simulink model "ANCbyFxLMS"  (R2024a)
settings: Solver=FixedStepDiscrete  StartTime=0.0  StopTime=1000000  RelTol=1e-3
settings Model: Creator=chenxinzhang  LastModifiedBy=chenxinzhang
settings SolverCC: AlgebraicLoopSolver=TrustRegion  AutoInsertRateTranBlk=on
settings DataIOCC: LimitDataPoints=on  SaveOutput=off  SignalLogging=off  SaveTime=off
settings OptimizationCC: LifeSpan=inf
settings DebuggingCC: AlgebraicLoopMsg=error  SingleTaskRateTransMsg=error  UnconnectedInputMsg=warning  UnconnectedOutputMsg=warning  UnconnectedLineMsg=warning  AllowSymbolicDim=off  SFUnexpectedBacktrackingDiag=warning  SFNoUnconditionalDefaultTransitionDiag=warning  SFExecutionAtInitializationDiag=none  ArithmeticOperatorsInVariantConditions=warning
settings ModelReferenceCC: EnableRefExpFcnMdlSchedulingChecks=on
settings SFSimCC: SimUseLocalCustomCode=off  CustomCodeUndefinedFunction=UseInterfaceOnly
settings RTWCC: RTWUseLocalCustomCode=off  GPUComputeCapability=3.5
settings CodeAppCC: StateflowObjectComments=on
settings GRTTargetCC: TargetLangStandard=C89/C90 (ANSI)
settings ConfigComp: CovMetricSettings=dw  CovSaveCumulativeToWorkspaceVar=on  CovSaveSingleToWorkspaceVar=on  CovExternalEMLEnable=off  CovSFcnEnable=off

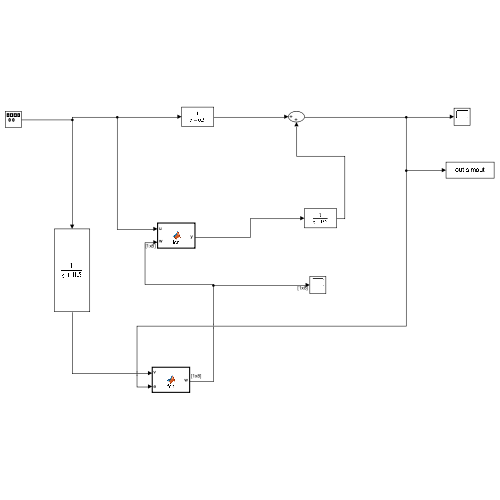
[thumbnail: Simulink's stored preview of the top-level diagram]
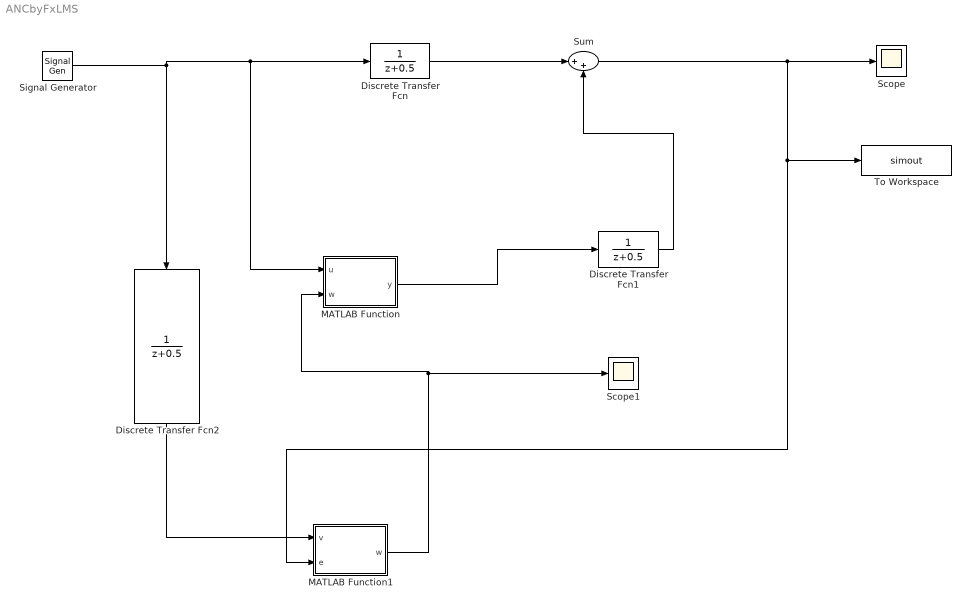
== system ANCbyFxLMS ==
  Discrete Transfer Fcn : DiscreteTransferFcn  Numerator=[0 1]
  Discrete Transfer Fcn1 : DiscreteTransferFcn  Numerator=[0 1]
  Discrete Transfer Fcn2 : DiscreteTransferFcn  Numerator=[0 1]
  MATLAB Function : MATLAB Function  TreatAsAtomicUnit=on
  MATLAB Function1 : MATLAB Function  TreatAsAtomicUnit=on
  Scope : Scope
  Scope1 : Scope
  Signal Generator : SignalGenerator  Frequency=10  Units=rad/sec
  Sum : Sum  Inputs=|++
  To Workspace : ToWorkspace  VariableName=simout  SaveFormat=Timeseries  SampleTime=-1
  wires:
  Signal Generator/1 -> Discrete Transfer Fcn2/1, MATLAB Function/1(u), Discrete Transfer Fcn/1
  Discrete Transfer Fcn/1 -> Sum/1
  Discrete Transfer Fcn1/1 -> Sum/2
  Sum/1 -> To Workspace/1, MATLAB Function1/2(e), Scope/1
  Discrete Transfer Fcn2/1 -> MATLAB Function1/1(v)
  MATLAB Function/1(y) -> Discrete Transfer Fcn1/1
  MATLAB Function1/1(w) -> Scope1/1, MATLAB Function/2(w)

== matlab function ANCbyFxLMS/MATLAB Function ==
  data: u input; y output; w input
function y = fcn(u, w)
%#codegen
persistent xbuf

if isempty(xbuf)
    xbuf = zeros(1,8);
end

xbuf(2:8) = xbuf(1:7);
xbuf(1) = u;

y = w * xbuf.';

if ~isfinite(y)
    y = 0;
elseif y > 1e3
    y = 1e3;
elseif y < -1e3
    y = -1e3;
end

== matlab function ANCbyFxLMS/MATLAB Function1 ==
  data: v input; w output; e input
function w = fcn(v, e)
%#codegen
persistent wbuf vbuf
mu = 1e-6;
if isempty(wbuf)
    wbuf = zeros(1,8);
end
if isempty(vbuf)
    vbuf = zeros(1,8);
end
vbuf(2:8) = vbuf(1:7);
vbuf(1) = v;
wbuf = wbuf - mu * e * vbuf;
for k = 1:8 
    if ~isfinite(wbuf(k))
        wbuf(k) = 0;
    elseif wbuf(k) > 10
        wbuf(k) = 10;
    elseif wbuf(k) < -10
        wbuf(k) = -10;
    end
end
w = wbuf;
